simulink model "Cau1"  (R2021b)
settings: Solver=VariableStepAuto  StartTime=0.0  StopTime=1  RelTol=1e-3
libraries: commdigbbndam3 x2, commfilt2 x2, commchan3 x1, commsink2 x1, commutil2 x1, commrandsrc3 x1
settings Model: Creator=ICTLAB  LastModifiedBy=ICTLAB

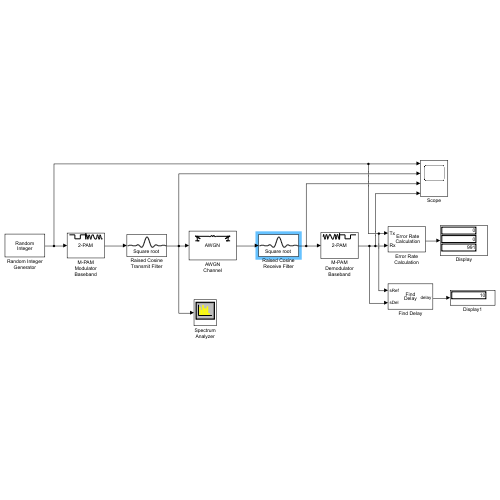
[thumbnail: Simulink's stored preview of the top-level diagram]
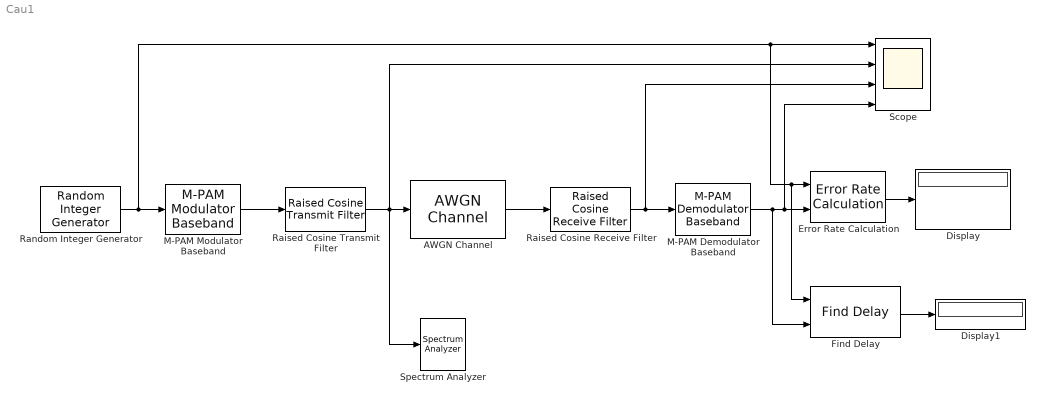
== system Cau1 ==
  AWGN Channel : commchan3/AWGN Channel  InputProcessing=Columns as channels (frame based)  seed=67  noiseMode="Signal to noise ratio  (Eb/No)"  EbNodB=10  EsNodB=10  SNRdB=10  bitsPerSym=1  Ps=1  Tsym=1/8000  variance=1
  Display : Display
  Display1 : Display
  Error Rate Calculation : commsink2/Error Rate Calculation  N=10  st_delay=0  cp_mode=Entire frame  subframe=[]  PMode=Port  WsName=ErrorVec  RsMode2=off  stop=off  numErr=100  maxBits=1e6
  Find Delay : commutil2/Find Delay  corrLength=200  chgSigOP=off  stopUpdate=off  numConstDelay=3
      settings: SourceProductBaseCode=CM
  M-PAM Demodulator Baseband : commdigbbndam3/M-PAM Demodulator Baseband  M=2  OutType=Integer  Dec=Gray  PowType=Min. distance between symbols  MinDist=2  AvgPow=1  PeakPow=1  outDtype1=Inherit via internal rule  outDtype2=Inherit via internal rule  denormFactorWordLen=16  denormFactorDataTypeStr=Inherit: Same word length as input  denormFactorLastDataTypeStr=Inherit: Same word length as input  prodOutWordLen=16  prodOutRoundingMode=Floor  prodOutOverflowMode=Wrap  prodOutOvFlMode=off  prodOutOvFlModeLastStrValue=off  sumWordLen=16
      settings: SourceProductBaseCode=CM
  M-PAM Modulator Baseband : commdigbbndam3/M-PAM Modulator Baseband  M=2  InType=Integer  Enc=Gray  PowType=Min. distance between symbols  MinDist=2  AvgPow=1  PeakPow=1  outDtype=double  outWordLen=16  outUDDataType=sfix(16)  outFracLenMode=Best precision  outFracLen=15  outDataTypeStr=double  outLastDataTypeStr=double
      settings: SourceProductBaseCode=CM
  Raised Cosine Receive Filter : commfilt2/Raised Cosine Receive Filter  filtType=Square root  R=1  filtSpan=10  N=8  downFactor=8  downOffset=0  filterGain=1  RateOptions=Allow multirate processing  framing=Mute  checkCoeff=off  variableName=rcRxFilt  currentFiltSpan=10  D=5  inputOffset=0  sampMode=Mute  saveAsFlag=0  rateMode=Downsampling  checkGain=Normalized  launchFVT=on  roundingMode=Floor  overflowMode=off  coeffDataTypeStr=Inherit: Same word length as input  coeffMin=[]  coeffMax=[]  coeffLastDataTypeStr=Inherit: Same word length as input  accumDataTypeStr=Inherit: Same as product output  accumLastDataTypeStr=Inherit: Same as product output  outputDataTypeStr=Inherit: Same as accumulator  outputMin=[]  outputMax=[]  outputLastDataTypeStr=Inherit: Same as accumulator
  Raised Cosine Transmit Filter : commfilt2/Raised Cosine Transmit Filter  filtType=Square root  R=1  filtSpan=10  N=8  filterGain=1  RateOptions=Allow multirate processing  framing=Mute  checkCoeff=off  variableName=rcTxFilt  checkGain=Normalized  sampMode=Mute  saveAsFlag=0  currentFiltSpan=10  D=5  launchFVT=on  roundingMode=Floor  overflowMode=off  coeffDataTypeStr=Inherit: Same word length as input  coeffMin=[]  coeffMax=[]  coeffLastDataTypeStr=Inherit: Same word length as input  outputDataTypeStr=Inherit: Same as accumulator  outputMin=[]  outputMax=[]  outputLastDataTypeStr=Inherit: Same as accumulator
  Random Integer Generator : commrandsrc3/Random Integer Generator  SetSize=2  SeedSource=Auto  Seed=0  SampleTime=1/1000  SamplesPerFrame=1  OutputDataType=double  SimulateUsing=Interpreted execution
  Scope : Scope  NumInputPorts=4
  Spectrum Analyzer : SpectrumAnalyzer
  wires:
  Random Integer Generator/1 -> Find Delay/1, Error Rate Calculation/1, Scope/1, M-PAM Modulator Baseband/1
  M-PAM Modulator Baseband/1 -> Raised Cosine Transmit Filter/1
  Raised Cosine Transmit Filter/1 -> Spectrum Analyzer/1, Scope/2, AWGN Channel/1
  AWGN Channel/1 -> Raised Cosine Receive Filter/1
  Raised Cosine Receive Filter/1 -> Scope/3, M-PAM Demodulator Baseband/1
  M-PAM Demodulator Baseband/1 -> Find Delay/2, Scope/4, Error Rate Calculation/2
  Error Rate Calculation/1 -> Display/1
  Find Delay/1 -> Display1/1
